simulink library "libslotcar"  (R2018b)
settings: Solver=VariableStepAuto  StartTime=0.0  StopTime=10.0  RelTol=1e-3
undefined symbols (not defined in the file): DiscIntNeverNeededParam, Discrete, Time
libraries: simulink x4, $bdroot x2, bbblueSensorLib x1, ctrlSharedLib x1
settings Model: Creator=Lenovo  LastModifiedBy=Lenovo
settings DebuggingCC: LibraryContextMissingDiagnostic=none
settings SFSimCC: SimUseLocalCustomCode=off
settings RTWCC: RTWUseLocalCustomCode=off

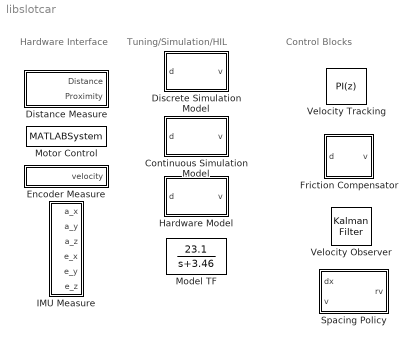
== system libslotcar ==
  note: Tuning/Simulation/HIL
  note: Hardware
      | Interface
  note: Control Blocks
  Continuous Simulation Model : Subsystem  mask{tsparam=-1, mparam=0.173, dparam=0.018, nparam=9/28, uparam=12.25-0.7, rparam=5, kparam=0.005, ksparam=0.7183, kdparam=0.3415}
      mask prompts: tsparam "Ts"; mparam "m"; dparam "d"; nparam "n"; uparam "U"; rparam "R"; kparam "k"; ksparam "ks"; kdparam "kd"
      mask DialogControl DescGroupVar Prompt: Car Model
      mask DialogControl DescTextVar Prompt: Simplified simulation model of slotcar dynamics
      mask DialogControl Container4 Prompt: Car
      mask DialogControl Container5 Prompt: Motor
      mask DialogControl Container3 Prompt: Friction
  Discrete Simulation Model : Subsystem  mask{tsparam=-1, mparam=0.173, dparam=0.018, nparam=9/28, uparam=12.25-0.7, rparam=5, kparam=0.005, ksparam=0.7183, kdparam=0.3415}
      mask prompts: tsparam "Ts"; mparam "m"; dparam "d"; nparam "n"; uparam "U"; rparam "R"; kparam "k"; ksparam "ks"; kdparam "kd"
      mask DialogControl DescGroupVar Prompt: Car Model
      mask DialogControl DescTextVar Prompt: Simplified simulation model of slotcar dynamics
      mask DialogControl Container4 Prompt: Car
      mask DialogControl Container5 Prompt: Motor
      mask DialogControl Container3 Prompt: Friction
  Distance Measure : Subsystem  mask{tc=0.016, margin=0.005}
      mask prompts: tc "Lowpass time constant"; margin "Distance margin"
      mask DialogControl DescGroupVar Prompt: Distance Measure (mask)
      mask DialogControl DescTextVar Prompt: Wraps the I2C proximity sensor and adds calculation of distance.
  Encoder Measure : Subsystem  mask{encts=1/400, encres=20, gearratio=9/28, diameter=0.0183, reversed=on}
      mask prompts: encts "Sample Time"; encres "Ticks per rotation"; gearratio "Gear ratio"; diameter "Wheel diameter"
  Friction Compensator : Subsystem  mask{coul=0.7183, visc=0.3415, Gain=1/3.9963}
      mask prompts: coul "Simulink:masks:CoulombFrictionValueOffset_MP"; visc "Simulink:masks:CoefficientOfViscousFrictionGain_MP"; Gain "Inverse of duty to linear force gain"
      mask TypeOptions coul:
      | Coulomb &
      | Viscous Friction/offset
      mask TypeOptions visc:
      | Coulomb &
      | Viscous Friction/gain
      mask TypeOptions Gain: Gain/Gain
      mask DialogControl Container3 Prompt: Friction
      mask DialogControl coul Prompt: Coulomb friction value (Offset):
      mask DialogControl visc Prompt: Coefficient of viscous friction (Gain):
      mask DialogControl Container5 Prompt: Gain
  Hardware Model : Subsystem  mask{freq=25000, SampleTime=1/400, encts=1/100, encres=20, gearratio=9/28, diameter=0.018, reversed=on}
      mask prompts: freq "PWM frequency:"; encts "Sample Time"; encres "Ticks per rotation"; gearratio "Gear ratio"; diameter "Wheel diameter"
      mask TypeOptions freq: Motor Control1/freq
      mask TypeOptions SampleTime: Motor Control1/SampleTime
      mask TypeOptions encts: Encoder Measure1/encts
      mask TypeOptions encres: Encoder Measure1/encres
      mask TypeOptions gearratio: Encoder Measure1/gearratio
      mask TypeOptions diameter: Encoder Measure1/diameter
      mask TypeOptions reversed: Encoder Measure1/reversed
      mask DialogControl Container3 Prompt: DC motor
      mask DialogControl Container4 Prompt: Encoder
  IMU Measure : Subsystem
  Model TF : TransferFcn  Numerator=23.1  Denominator=[1 3.46]  ContinuousStateAttributes='velocity'
  Motor Control : MATLABSystem  System=slotcar.Motor.MotorSysObject  freq=25000  SampleTime=0.1
      mask Type: slotcar.Motor.MotorSysObject
      mask Display:
      | disp('DC');
      | port_label('input',1,'duty');
  Spacing Policy : Subsystem  mask{Gain=400, dcor=0.01, h0=0.05, hv=0.05}
      mask prompts: Gain "Aggresiveness:"; dcor "Corridor length:"; h0 "Constant headway:"; hv "Speed headway:"
      mask TypeOptions Gain: Gain/Gain
      mask TypeOptions dcor: Spacing Error/dcor
      mask TypeOptions h0: Spacing Error/h0
      mask TypeOptions hv: Spacing Error/hv
  Velocity Observer : ctrlSharedLib/Kalman Filter  TimeDomain=Discrete-Time  UseCurrentEstimator=on  ModelSource=Individual A, B, C, D matrices  ModelSourceVariable=ss(0.95,1,1,1,0)  A=-3.46  B=23.1  C=1  D=0  NumberOfStates=1  NumberOfInputs=1  NumberOfOutputs=1  InitialEstimateSource=Dialog  X0=0  P0=10  UseK=off  UseGH=off  NumberOfProcessNoiseInputs=1  G=1  TimeInvariantG=on  H=0  TimeInvariantH=on  Q=0.5  TimeInvariantQ=on  R=1  TimeInvariantR=on  N=0  TimeInvariantN=on  AddInputPort=on  AddEnablePort=off  OutputEstimatedY=off  OutputP=off  Ts=1/400
      settings: SourceProductBaseCode=CT
  Velocity Tracking : simulink/Continuous/PID Controller  Controller=PI  Form=Parallel  TimeDomain=Discrete-time  SampleTime=-1  IntegratorMethod=Forward Euler  FilterMethod=Forward Euler  ControllerParametersSource=internal  P=0.202863589993018  I=2.14911342042457  D=0  UseFilter=on  N=100  TunerSelectOption=Transfer Function Based (PID Tuner App)  InitialConditionSource=internal  InitialConditionForIntegrator=0  InitialConditionForFilter=0  DifferentiatorICPrevScaledInput=0  ExternalReset=none  TrackingMode=off  Kt=1  LimitOutput=on  UpperSaturationLimit=0.4  LowerSaturationLimit=-0.4  LinearizeAsGain=off  AntiWindupMode=clamping  Kb=1  POutMin=[]  POutMax=[]  IOutMin=[]  IOutMax=[]  DOutMin=[]  DOutMax=[]  NOutMin=[]  NOutMax=[]  SumOutMin=[]  SumOutMax=[]  SaturationOutMin=[]  SaturationOutMax=[]  PParamMin=[]  PParamMax=[]  IParamMin=[]  IParamMax=[]  DParamMin=[]  DParamMax=[]  NParamMin=[]  NParamMax=[]  KbParamMin=[]  KbParamMax=[]  KtParamMin=[]  KtParamMax=[]  KbOutMin=[]  KbOutMax=[]  KtOutMin=[]  KtOutMax=[]  IntegratorOutMin=[]  IntegratorOutMax=[]  FilterOutMin=[]  FilterOutMax=[]  SumI1OutMin=[]  SumI1OutMax=[]  SumI2OutMin=[]  SumI2OutMax=[]  SumI3OutMin=[]  SumI3OutMax=[]  SumI4OutMin=[]  SumI4OutMax=[]  SumDOutMin=[]  SumDOutMax=[]  DifferentiatorOutMin=[]  DifferentiatorOutMax=[]  FilterDiffOutCoefMin=[]  FilterDiffOutCoefMax=[]  ReciprocalOutMin=[]  ReciprocalOutMax=[]  SumDenOutMin=[]  SumDenOutMax=[]  SumNumOutMin=[]  SumNumOutMax=[]  DivideOutMin=[]  DivideOutMax=[]  IntegratorContinuousStateAttributes=''  IntegratorStateMustResolveToSignalObject=off  IntegratorRTWStateStorageClass=Auto  FilterContinuousStateAttributes=''  FilterStateMustResolveToSignalObject=off  FilterRTWStateStorageClass=Auto  ParallelPVariant=InternalParameters  IdealPVariant=Disabled  IVariant=InternalParameters  DVariant=Disabled  IntegratorVariant=Discrete  SatVariant=Enabled  AWVariant=DiscClampingParallel  PCopyVariant=Disabled  TRVariant=Disabled  FdbkBlocksVariant=Forward  IdealPFdbkVariant=Disabled  SatFdbkVariant=Disabled  DerivativeFilterVariant=Disabled  NVariant=Disabled  NCopyVariant=Disabled_SignalSpec  FilterICVariant=Disabled  IntegratorICVariant=InternalICs  ExternalResetVariant=Disabled  TRSumVariant=Passthrough  SumFdbkVariant=Disabled  SumVariant=Sum_PI

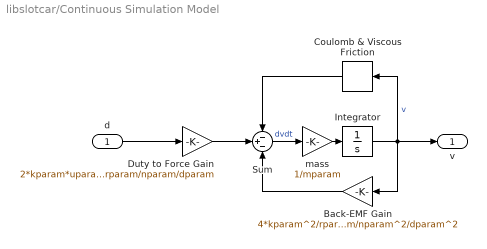
== system libslotcar/Continuous Simulation Model ==
  d : Inport
  Back-EMF Gain : Gain  Gain=4*kparam^2/rparam/nparam^2/dparam^2
  Coulomb & Viscous Friction : simulink/Discontinuities/Coulomb & Viscous Friction  offset=ksparam  gain=kdparam
      settings: SourceProductName=Simulink
  Duty to Force Gain : Gain  Gain=2*kparam*uparam/rparam/nparam/dparam
  Integrator : Integrator
  Sum : Sum  Inputs=-+-
  mass : Gain  Gain=1/mparam
  v : Outport
  wires:
  Sum/1 -> mass/1  "dvdt"
  Integrator/1 -> Back-EMF Gain/1, Coulomb & Viscous Friction/1, v/1  "v"
  Duty to Force Gain/1 -> Sum/2
  Back-EMF Gain/1 -> Sum/3
  d/1 -> Duty to Force Gain/1
  Coulomb & Viscous Friction/1 -> Sum/1
  mass/1 -> Integrator/1

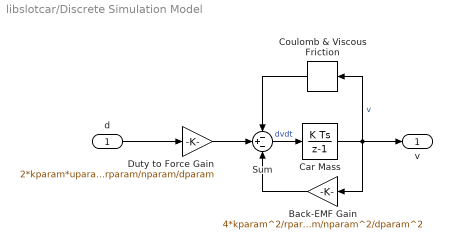
== system libslotcar/Discrete Simulation Model ==
  d : Inport
  Back-EMF Gain : Gain  Gain=4*kparam^2/rparam/nparam^2/dparam^2
  Car Mass : DiscreteIntegrator  gainval=1/mparam  SampleTime=tsparam  UpperSaturationLimit=30  LowerSaturationLimit=-30  ICPrevOutput=DiscIntNeverNeededParam  ICPrevScaledInput=DiscIntNeverNeededParam
  Coulomb & Viscous Friction : simulink/Discontinuities/Coulomb & Viscous Friction  offset=ksparam  gain=kdparam
      settings: SourceProductName=Simulink
  Duty to Force Gain : Gain  Gain=2*kparam*uparam/rparam/nparam/dparam
  Sum : Sum  Inputs=-+-
  v : Outport
  wires:
  Sum/1 -> Car Mass/1  "dvdt"
  Car Mass/1 -> Back-EMF Gain/1, Coulomb & Viscous Friction/1, v/1  "v"
  Duty to Force Gain/1 -> Sum/2
  Back-EMF Gain/1 -> Sum/3
  d/1 -> Duty to Force Gain/1
  Coulomb & Viscous Friction/1 -> Sum/1

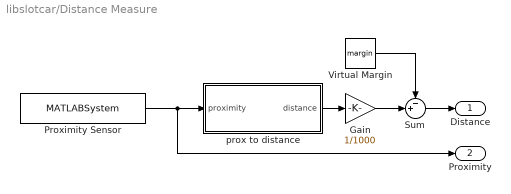
== system libslotcar/Distance Measure ==
  Gain : Gain  Gain=1/1000
  Proximity Sensor : MATLABSystem  System=slotcar.ProximityI2C.ProximitySysObject  TC=tc  SampleTime=1/400
      mask Type: slotcar.ProximityI2C.ProximitySysObject
      mask Display:
      | disp('VCNL4010');
      | port_label('output',1,'prox');
  Sum : Sum  Inputs=-+|
  Virtual Margin : Constant  Value=margin
  "prox to distance " : MATLAB Function  TreatAsAtomicUnit=on
  Distance : Outport
  Proximity : Outport  Port=2
  wires:
  Proximity Sensor/1 -> Proximity/1, "prox to distance "/1(proximity)
  "prox to distance "/1(distance) -> Gain/1
  Sum/1 -> Distance/1
  Virtual Margin/1 -> Sum/1
  Gain/1 -> Sum/2

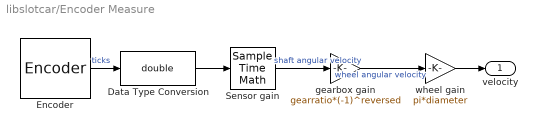
== system libslotcar/Encoder Measure ==
  Data Type Conversion : DataTypeConversion  OutDataTypeStr=double  RndMeth=Nearest
  Encoder : bbblueSensorLib/Encoder  Channel=1  Mode=Reset at each Sample time  SampleTime=encts  SimulateUsing=Code generation
      settings: SourceProductName=Simulink Coder Support Package for BeagleBone Blue Hardware
  Sensor gain : SampleTimeMath  TsampMathOp=/  weightValue=encres  TsampMathImp=Offline Scaling Adjustment
  gearbox gain : Gain  Gain=gearratio*(-1)^reversed
  wheel gain : Gain  Gain=pi*diameter  OutDataTypeStr=double
  velocity : Outport
  wires:
  Encoder/1 -> Data Type Conversion/1  "ticks"
  Sensor gain/1 -> gearbox gain/1  "shaft angular velocity"
  gearbox gain/1 -> wheel gain/1  "wheel angular velocity"
  wheel gain/1 -> velocity/1
  Data Type Conversion/1 -> Sensor gain/1

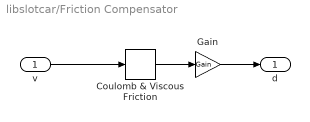
== system libslotcar/Friction Compensator ==
  v : Inport
  Coulomb & Viscous Friction : simulink/Discontinuities/Coulomb & Viscous Friction  offset=coul  gain=visc
      settings: SourceProductName=Simulink
  Gain : Gain  Gain=Gain
  d : Outport
  wires:
  Coulomb & Viscous Friction/1 -> Gain/1
  v/1 -> Coulomb & Viscous Friction/1
  Gain/1 -> d/1

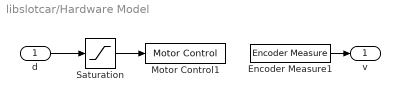
== system libslotcar/Hardware Model ==
  d : Inport
  Encoder Measure1 : $bdroot/Encoder Measure  encts=encts  encres=encres  gearratio=gearratio  diameter=diameter  reversed=on
  Motor Control1 : $bdroot/Motor Control  freq=freq  SampleTime=SampleTime
  Saturation : Saturate  UpperLimit=0.4  LowerLimit=-0.4
  v : Outport
  wires:
  Encoder Measure1/1 -> v/1
  d/1 -> Saturation/1
  Saturation/1 -> Motor Control1/1

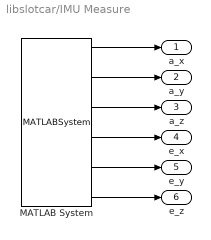
== system libslotcar/IMU Measure ==
  MATLAB System : MATLABSystem  System=slotcar.IMU.ImuSysObject  SampleTime=-1
      mask Type: slotcar.IMU.ImuSysObject
      mask Display: disp(['IMU' char(10) 'Voltages']);
  a_x : Outport
  a_y : Outport  Port=2
  a_z : Outport  Port=3
  e_x : Outport  Port=4
  e_y : Outport  Port=5
  "e_z " : Outport  Port=6
  wires:
  MATLAB System/4 -> e_x/1
  MATLAB System/2 -> a_y/1
  MATLAB System/1 -> a_x/1
  MATLAB System/3 -> a_z/1
  MATLAB System/6 -> "e_z "/1
  MATLAB System/5 -> e_y/1

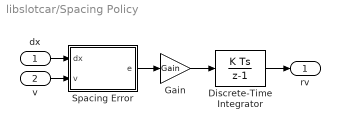
== system libslotcar/Spacing Policy ==
  dx : Inport
  v : Inport  Port=2
  Discrete-Time Integrator : DiscreteIntegrator  gainval=200  SampleTime=-1  LimitOutput=on  UpperSaturationLimit=0.8  LowerSaturationLimit=-0.2  ICPrevOutput=DiscIntNeverNeededParam  ICPrevScaledInput=DiscIntNeverNeededParam
  Gain : Gain  Gain=Gain
  Spacing Error : MATLAB Function  TreatAsAtomicUnit=on  mask{dcor=dcor, h0=h0, hv=hv}
      mask prompts: dcor "Corridor length:"; h0 "Constant headway:"; hv "Speed headway:"
  rv : Outport
  wires:
  Spacing Error/1(e) -> Gain/1
  dx/1 -> Spacing Error/1(dx)
  v/1 -> Spacing Error/2(v)
  Discrete-Time Integrator/1 -> rv/1
  Gain/1 -> Discrete-Time Integrator/1

== matlab function libslotcar/Spacing Policy/Spacing Error ==
  data: dx input size=1; e output size=1; v input size=1; h0 parameter size=1; hv parameter size=1; dcor parameter size=1
function e = fcn(dx, v, h0, hv, dcor)
xmin = h0 + hv * v;
xmax = xmin + dcor;
if dx < xmin
    e = dx - xmin;
elseif dx > xmax
    e = dx - xmax;
else
    e = 0;
end

== matlab function libslotcar/Distance Measure/prox to distance  ==
  data: proximity input; distance output
function distance = fcn(proximity)
    proximity = double(proximity);
    if proximity<=28.5
        distance = 10*(14.14*exp(-0.2527*proximity)+17.04*exp(-0.01403*proximity));
        if distance>250
            distance = 250;
        end    
    elseif proximity>28.5&&proximity<=467.5
        distance = 10*(7.244*exp(-0.0233*proximity)+7.959*exp(-0.001185*proximity));
    else
        distance = 10*(3.749*exp(-0.0008848*proximity)+2.124*exp(-2.946e-05*proximity));        
    end
end
